simulink subsystem "INBOUND_MSG_UNMAP"  (R2023a)
settings: Solver=VariableStepAuto  StartTime=0.0  StopTime=10.0  RelTol=1e-3
undefined symbols (not defined in the file or in its folder): ARMED, FLIGHT_MODE, Sticks
libraries: aerolibutil x3, sharedtransform x1
settings Model: Creator=thesa  LastModifiedBy=yzk0058

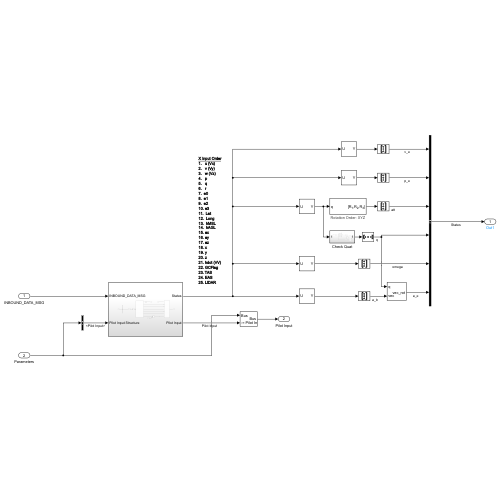
[thumbnail: Simulink's stored preview of the top-level diagram]
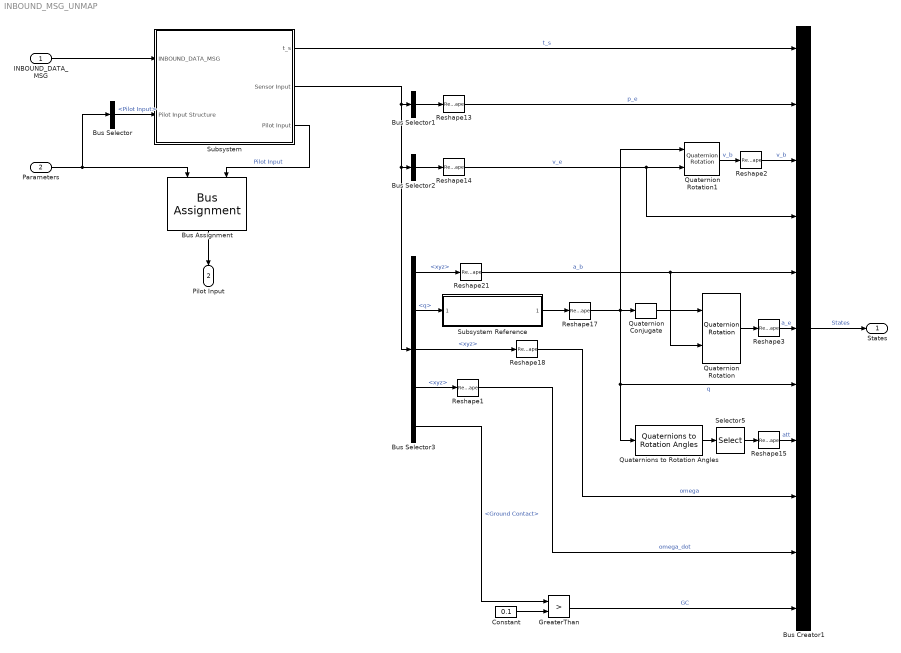
== system INBOUND_MSG_UNMAP ==
  INBOUND_DATA_MSG : Inport
  Parameters : Inport  Port=2
  Bus Assignment : BusAssignment  AssignedSignals=Pilot Input
  Bus Creator1 : BusCreator  Inputs=11
  Bus Selector : BusSelector  OutputSignals=Pilot Input
  Bus Selector1 : BusSelector  OutputSignals=vehicle local position.x,vehicle local position.y,vehicle local position.z  OutputAsBus=on
  Bus Selector2 : BusSelector  OutputSignals=vehicle local position.vx,vehicle local position.vy,vehicle local position.vz  OutputAsBus=on
  Bus Selector3 : BusSelector  OutputSignals=vehicle acceleration.xyz,vehicle attitude.q,vehicle angular velocity.xyz,vehicle angular acceleration.xyz,Ground Contact
  Constant : Constant  Value=0.1  OutDataTypeStr=Inherit: Inherit via back propagation
  GreaterThan : RelationalOperator  Operator=>  OutDataTypeStr=boolean  RndMeth=Simplest  InputSameDT=off
  Quaternion Conjugate : aerolibutil/Quaternion Conjugate
  Quaternion Rotation : aerolibutil/Quaternion Rotation
  Quaternion Rotation1 : aerolibutil/Quaternion Rotation
  Quaternions to Rotation Angles : sharedtransform/Quaternions to Rotation Angles  rotationOrder=ZYX  aMode=aMode
  Reshape{1..3,13..15,18,21} (8 alike) : Reshape  OutputDimensionality=Column vector (2-D)
  Reshape17 : Reshape  OutputDimensionality=Row vector (2-D)
  Selector5 : Selector  InputPortWidth=3  IndexOptions=Index vector (dialog)  Indices=[3,2,1]  OutputSizes=1
  Subsystem : Subsystem
  Subsystem Reference : Subsystem  ReferencedSubsystem=Check_Quat
  States : Outport
  Pilot Input : Outport  Port=2
  wires:
  Subsystem Reference/1 -> Reshape17/1
  Bus Selector/1 -> Subsystem/2(Pilot Input Structure)  "<Pilot Input>"
  Parameters/1 -> Bus Assignment/1, Bus Selector/1
  Bus Creator1/1 -> States/1  "States"
  Reshape15/1 -> Bus Creator1/8  "att"
  Reshape13/1 -> Bus Creator1/2  "p_e"
  Reshape14/1 -> Quaternion Rotation1/2, Bus Creator1/4  "v_e"
  Reshape17/1 -> Quaternion Conjugate/1, Quaternion Rotation1/1, Bus Creator1/7, Quaternions to Rotation Angles/1  "q"
  Reshape18/1 -> Bus Creator1/9  "omega"
  Quaternions to Rotation Angles/1 -> Selector5/1
  Bus Selector1/1 -> Reshape13/1
  Bus Selector2/1 -> Reshape14/1
  Quaternion Rotation/1 -> Reshape3/1
  Bus Selector3/1 -> Reshape21/1  "<xyz>"
  Reshape21/1 -> Quaternion Rotation/2, Bus Creator1/5  "a_b"
  Bus Assignment/1 -> Pilot Input/1
  Subsystem/3(Pilot Input) -> Bus Assignment/2  "Pilot Input"
  INBOUND_DATA_MSG/1 -> Subsystem/1(INBOUND_DATA_MSG)
  Bus Selector3/3 -> Reshape18/1  "<xyz>"
  Bus Selector3/2 -> Subsystem Reference/1  "<q>"
  Selector5/1 -> Reshape15/1
  Quaternion Rotation1/1 -> Reshape2/1  "v_b"
  Bus Selector3/4 -> Reshape1/1  "<xyz>"
  Reshape1/1 -> Bus Creator1/10  "omega_dot"
  Subsystem/1(t_s) -> Bus Creator1/1  "t_s"
  Reshape2/1 -> Bus Creator1/3  "v_b"
  Reshape3/1 -> Bus Creator1/6  "a_e"
  Quaternion Conjugate/1 -> Quaternion Rotation/1
  GreaterThan/1 -> Bus Creator1/11  "GC"
  Subsystem/2(Sensor Input) -> Bus Selector1/1, Bus Selector2/1, Bus Selector3/1
  Constant/1 -> GreaterThan/2
  Bus Selector3/5 -> GreaterThan/1  "<Ground Contact>"

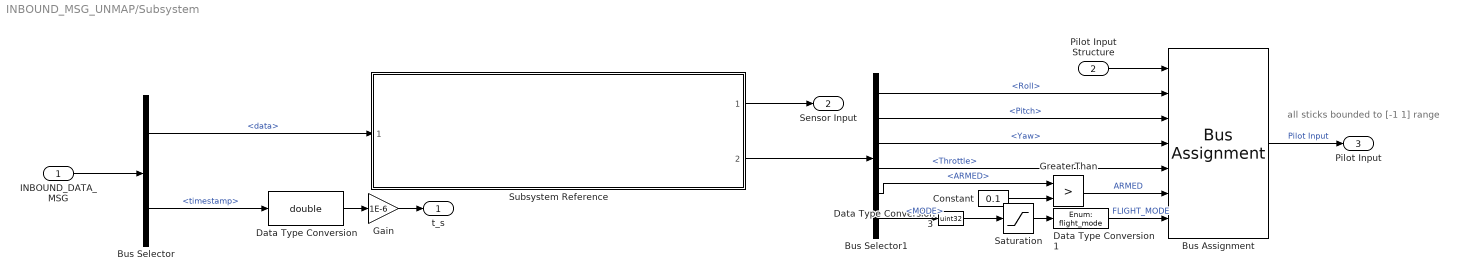
== system INBOUND_MSG_UNMAP/Subsystem ==
  note: all sticks bounded to [-1 1] range
  INBOUND_DATA_MSG : Inport
  Pilot Input Structure : Inport  Port=2
  Bus Assignment : BusAssignment  AssignedSignals=Sticks.roll_stick,Sticks.pitch_stick,Sticks.yaw_stick,Sticks.Throttle_stick,ARMED,FLIGHT_MODE
  Bus Selector : BusSelector  OutputSignals=data,timestamp
  Bus Selector1 : BusSelector  OutputSignals=Roll,Pitch,Yaw,Throttle,ARMED,MODE
  Constant : Constant  Value=0.1  OutDataTypeStr=Inherit: Inherit via back propagation
  Data Type Conversion : DataTypeConversion  OutDataTypeStr=double  SaturateOnIntegerOverflow=off  RndMeth=Floor
  Data Type Conversion1 : DataTypeConversion  OutDataTypeStr=Enum: flight_mode  SaturateOnIntegerOverflow=off  RndMeth=Floor
  Data Type Conversion3 : DataTypeConversion  OutDataTypeStr=uint32  SaturateOnIntegerOverflow=off  RndMeth=Floor
  Gain : Gain  Gain=1E-6
  GreaterThan : RelationalOperator  Operator=>  OutDataTypeStr=boolean  RndMeth=Simplest  InputSameDT=off
  Saturation : Saturate  UpperLimit=8  LowerLimit=0
  Subsystem Reference : Subsystem  ReferencedSubsystem=sm_inbound_interpreter
  t_s : Outport
  Sensor Input : Outport  Port=2
  Pilot Input : Outport  Port=3
  wires:
  Saturation/1 -> Data Type Conversion1/1
  Data Type Conversion3/1 -> Saturation/1
  Bus Selector1/6 -> Data Type Conversion3/1  "<MODE>"
  Subsystem Reference/2 -> Bus Selector1/1
  Subsystem Reference/1 -> Sensor Input/1
  Bus Selector/2 -> Data Type Conversion/1  "<timestamp>"
  Bus Selector/1 -> Subsystem Reference/1  "<data>"
  Gain/1 -> t_s/1
  Data Type Conversion/1 -> Gain/1
  INBOUND_DATA_MSG/1 -> Bus Selector/1
  Bus Assignment/1 -> Pilot Input/1  "Pilot Input"
  Bus Selector1/4 -> Bus Assignment/5  "<Throttle>"
  Bus Selector1/3 -> Bus Assignment/4  "<Yaw>"
  Bus Selector1/1 -> Bus Assignment/2  "<Roll>"
  GreaterThan/1 -> Bus Assignment/6  "ARMED"
  Bus Selector1/2 -> Bus Assignment/3  "<Pitch>"
  Constant/1 -> GreaterThan/2
  Data Type Conversion1/1 -> Bus Assignment/7  "FLIGHT_MODE"
  Bus Selector1/5 -> GreaterThan/1  "<ARMED>"
  Pilot Input Structure/1 -> Bus Assignment/1
